simulink model "Sim_tanksmodel_FGS"  (R2020b)
settings: Solver=FixedStepAuto  StartTime=0.0  StopTime=4000  FixedStep=1  RelTol=1e-3  EnableMultiTasking=on
InitFcn:
  | cd ..
  | cd ..
  | 
  | addpath(genpath('Controlador GS-PID'))
  | cd 'Controlador GS-PID\General'
  | inParameters
StopFcn:
  | BestGains1 = [AS(1).Kp AS(1).Ki AS(1).Kd];
  | BestGains2 = [AS(2).Kp AS(2).Ki AS(2).Kd];
  | BestGains3 = [AS(3).Kp AS(3).Ki AS(3).Kd];
  | save('deletetoreset.mat','BestGains1','BestGains2','BestGains3')
  | 
  | BestGains1 = SA(1).BestSol.Gain;
  | BestGains2 = SA(2).BestSol.Gain;
  | BestGains3 = SA(3).BestSol.Gain;
  | save('reset.mat','BestGains1','BestGains2','BestGains3')
undefined symbols (not defined in the file or in its folder): AS, he1, he2, Kd1, Kd2, Kd3, Ki1, Ki2, Ki3, Kp1, Kp2, Kp3, SA, Ts
libraries: simulink x4, pid_lib x1
settings Model: SimulationMode=accelerator  Creator=sahandar  LastModifiedBy=Usuario
settings SolverCC: AlgebraicLoopSolver=LineSearch
settings DataIOCC: LimitDataPoints=on  SaveFormat=Array  ReturnWorkspaceOutputs=off
settings OptimizationCC: LifeSpan=inf
settings DebuggingCC: AllowSymbolicDim=off  SFUnexpectedBacktrackingDiag=warning  SFNoUnconditionalDefaultTransitionDiag=warning  SFExecutionAtInitializationDiag=none  ArithmeticOperatorsInVariantConditions=warning
settings HardwareCC: ProdBitPerPointer=32  ProdBitPerSizeT=32  ProdBitPerPtrDiffT=32  ProdLargestAtomicFloat=None  ProdIntDivRoundTo=Undefined  ProdEndianess=Unspecified  ProdWordSize=32  ProdHWDeviceType=32-bit Generic
settings ModelReferenceCC: PropagateSignalLabelsOutOfModel=off
settings SFSimCC: SimUseLocalCustomCode=off  CustomCodeUndefinedFunction=UseInterfaceOnly
settings RTWCC: RTWUseLocalCustomCode=off
settings CodeAppCC: StateflowObjectComments=on
settings GRTTargetCC: TargetLangStandard=C89/C90 (ANSI)
settings ConfigComp: CovMetricSettings=dw  CovSaveCumulativeToWorkspaceVar=on  CovSaveSingleToWorkspaceVar=on  CovExternalEMLEnable=off

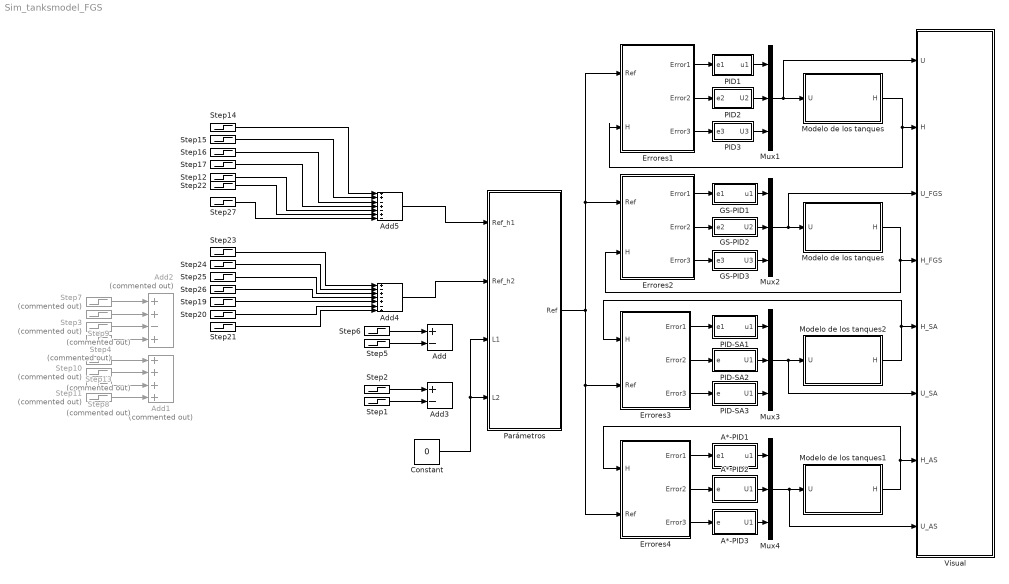
== system Sim_tanksmodel_FGS ==
  A*-PID1 : Subsystem
  A*-PID2 : Subsystem
  A*-PID3 : Subsystem
  Add : Sum  Inputs=+-
  Add1 : Sum  Commented=on  Inputs=++++
  Add2 : Sum  Commented=on  Inputs=++-+
  Add3 : Sum  Inputs=+-
  Add4 : Sum  Inputs=+-+-+-+
  Add5 : Sum  Inputs=++-+-+-
  Constant : Constant  Value=0
  Errores1 : Subsystem
  Errores2 : Subsystem
  Errores3 : Subsystem
  Errores4 : Subsystem
  GS-PID1 : Subsystem
  GS-PID2 : Subsystem
  GS-PID3 : Subsystem
  Modelo de los tanques : Subsystem
  "Modelo de los tanques " : Subsystem
  Modelo de los tanques1 : Subsystem
  Modelo de los tanques2 : Subsystem
  Mux{1..4} (4 alike) : Mux  Inputs=3
  PID-SA1 : Subsystem
  PID-SA2 : Subsystem
  PID-SA3 : Subsystem
  PID1 : Subsystem
  PID2 : Subsystem
  PID3 : Subsystem
  Parámetros : Subsystem
  Step1 : Step  Time=900  SampleTime=Ts
  Step10 : Step  Commented=on  Time=350  After=-0.03  SampleTime=Ts
  Step11 : Step  Commented=on  Time=1100  After=-0.03  SampleTime=Ts
  Step12 : Step  Time=2000  After=0.06  SampleTime=Ts
  Step13 : Step  Commented=on  Time=0  Before=he2  After=0.05  SampleTime=Ts
  Step14 : Step  Time=0  Before=he1  After=0.02  SampleTime=Ts
  Step15 : Step  Time=500  After=0.06  SampleTime=Ts
  Step16 : Step  Time=1000  After=0.06  SampleTime=Ts
  Step17 : Step  Time=1500  After=0.06  SampleTime=Ts
  Step19 : Step  Time=2000  After=0.06  SampleTime=Ts
  Step2 : Step  Time=800  SampleTime=Ts
  Step20 : Step  Time=2500  After=0.06  SampleTime=Ts
  Step21 : Step  Time=3000  After=0.06  SampleTime=Ts
  Step22 : Step  Time=2500  After=0.06  SampleTime=Ts
  Step23 : Step  Time=0  Before=he1  After=0.08  SampleTime=Ts
  Step24 : Step  Time=500  After=0.06  SampleTime=Ts
  Step25 : Step  Time=1000  After=0.06  SampleTime=Ts
  Step26 : Step  Time=1500  After=0.06  SampleTime=Ts
  Step27 : Step  Time=3000  After=0.06  SampleTime=Ts
  Step3 : Step  Commented=on  Time=700  After=0.05  SampleTime=Ts
  Step4 : Step  Commented=on  Time=1100  After=0.05  SampleTime=Ts
  Step5 : Step  Time=800  SampleTime=Ts
  Step6 : Step  Time=600  SampleTime=Ts
  Step7 : Step  Commented=on  Time=0  Before=he1  After=0.15  SampleTime=Ts
  Step8 : Step  Commented=on  Time=700  After=0.02  SampleTime=Ts
  Step9 : Step  Commented=on  Time=350  After=0.05  SampleTime=Ts
  Visual : Subsystem
  wires:
  Mux1/1 -> Modelo de los tanques/1(U), Visual/1(U)
  Modelo de los tanques/1(H) -> Errores1/2(H), Visual/2(H)
  GS-PID3/1(U3) -> Mux2/3
  Errores2/3(Error3) -> GS-PID3/1(e3)
  GS-PID2/1(U2) -> Mux2/2
  Errores2/2(Error2) -> GS-PID2/1(e2)
  GS-PID1/1(u1) -> Mux2/1
  Errores2/1(Error1) -> GS-PID1/1(e1)
  "Modelo de los tanques "/1(H) -> Errores2/2(H), Visual/4(H_FGS)
  Mux2/1 -> Visual/3(U_FGS), "Modelo de los tanques "/1(U)
  PID2/1(U2) -> Mux1/2
  PID3/1(U3) -> Mux1/3
  Errores1/2(Error2) -> PID2/1(e2)
  Errores1/3(Error3) -> PID3/1(e3)
  Errores1/1(Error1) -> PID1/1(e1)
  PID1/1(u1) -> Mux1/1
  PID-SA3/1(U1) -> Mux3/3
  PID-SA2/1(U1) -> Mux3/2
  Modelo de los tanques2/1(H) -> Errores3/1(H), Visual/5(H_SA)
  PID-SA1/1(u1) -> Mux3/1
  Errores3/3(Error3) -> PID-SA3/1(e)
  Errores3/1(Error1) -> PID-SA1/1(e1)
  Errores3/2(Error2) -> PID-SA2/1(e)
  Mux3/1 -> Visual/6(U_SA), Modelo de los tanques2/1(U)
  A*-PID3/1(U1) -> Mux4/3
  Parámetros/1(Ref) -> Errores1/1(Ref), Errores2/1(Ref), Errores3/2(Ref), Errores4/2(Ref)
  A*-PID2/1(U1) -> Mux4/2
  Errores4/2(Error2) -> A*-PID2/1(e)
  A*-PID1/1(u1) -> Mux4/1
  Errores4/3(Error3) -> A*-PID3/1(e)
  Modelo de los tanques1/1(H) -> Errores4/1(H), Visual/7(H_AS)
  Mux4/1 -> Modelo de los tanques1/1(U), Visual/8(U_AS)
  Errores4/1(Error1) -> A*-PID1/1(e1)
  Step3/1 -> Add2/3
  Step8/1 -> Add1/3
  Step9/1 -> Add2/2
  Step4/1 -> Add2/4
  Step7/1 -> Add2/1
  Step13/1 -> Add1/1
  Step11/1 -> Add1/4
  Step5/1 -> Add/2
  Step1/1 -> Add3/2
  Step10/1 -> Add1/2
  Step6/1 -> Add/1
  Step2/1 -> Add3/1
  Constant/1 -> Parámetros/4(L2), Parámetros/3(L1)
  Step24/1 -> Add4/2
  Step26/1 -> Add4/4
  Step19/1 -> Add4/5
  Step25/1 -> Add4/3
  Step14/1 -> Add5/1
  Step27/1 -> Add5/7
  Step23/1 -> Add4/1
  Step17/1 -> Add5/4
  Step20/1 -> Add4/6
  Step12/1 -> Add5/5
  Step22/1 -> Add5/6
  Step21/1 -> Add4/7
  Step16/1 -> Add5/3
  Step15/1 -> Add5/2
  Add5/1 -> Parámetros/1(Ref_h1)
  Add4/1 -> Parámetros/2(Ref_h2)

== system Sim_tanksmodel_FGS/A*-PID1 ==
  e1 : Inport
  Demux : Demux  Outputs=3
  Mux : Mux
  PID Controller : Subsystem
  S-Function : S-Function  FunctionName=sfun_Astar  Parameters=AS_vars1  SFunctionDeploymentMode=off  EnableBusSupport=off
  Saturation1 : Saturate  UpperLimit=1  LowerLimit=0
  Subsystem : Subsystem
  u1 : Outport
  wires:
  Saturation1/1 -> u1/1
  PID Controller/1(u) -> Saturation1/1
  Mux/1 -> S-Function/1
  Subsystem/1(ref) -> Mux/2
  Subsystem/2(enable) -> Mux/3
  S-Function/1 -> Demux/1
  Demux/3 -> PID Controller/4(Kd)  "Kd"
  e1/1 -> PID Controller/1(e), Mux/1
  Subsystem/3(iter) -> Mux/4
  Demux/1 -> PID Controller/2(Kp)  "Kp"
  Demux/2 -> PID Controller/3(Ki)  "Ki"

== system Sim_tanksmodel_FGS/A*-PID2 ==
  e : Inport
  Demux : Demux  Outputs=3
  Mux : Mux
  PID Controller : Subsystem
  S-Function : S-Function  FunctionName=sfun_Astar  Parameters=AS_vars2  SFunctionDeploymentMode=off  EnableBusSupport=off
  Saturation1 : Saturate  UpperLimit=1  LowerLimit=0
  Scope : Scope  NumInputPorts=3
  Subsystem : Subsystem
  U1 : Outport
  wires:
  Demux/2 -> PID Controller/3(Ki), Scope/2  "Ki"
  Demux/1 -> PID Controller/2(Kp), Scope/1  "Kp"
  Subsystem/3(iter) -> Mux/4
  e/1 -> PID Controller/1(e), Mux/1
  Demux/3 -> PID Controller/4(Kd), Scope/3  "Kd"
  S-Function/1 -> Demux/1
  Subsystem/2(enable) -> Mux/3
  Subsystem/1(ref) -> Mux/2
  Mux/1 -> S-Function/1
  Saturation1/1 -> U1/1
  PID Controller/1(u) -> Saturation1/1

== system Sim_tanksmodel_FGS/A*-PID3 ==
  e : Inport
  Demux : Demux  Outputs=3
  Gain : Gain  Gain=-1
  Mux : Mux
  PID Controller : Subsystem
  S-Function : S-Function  FunctionName=sfun_Astar  Parameters=AS_vars3  SFunctionDeploymentMode=off  EnableBusSupport=off
  Saturation1 : Saturate  UpperLimit=1  LowerLimit=0
  Scope : Scope  NumInputPorts=3
  Subsystem : Subsystem
  U1 : Outport
  wires:
  Saturation1/1 -> U1/1
  Mux/1 -> S-Function/1
  Subsystem/1(ref) -> Mux/2
  Subsystem/2(enable) -> Mux/3
  S-Function/1 -> Demux/1
  Demux/3 -> Scope/3, PID Controller/4(Kd)  "Kd"
  e/1 -> Mux/1, PID Controller/1(e)
  Subsystem/3(iter) -> Mux/4
  Demux/1 -> Scope/1, PID Controller/2(Kp)  "Kp"
  Demux/2 -> Scope/2, PID Controller/3(Ki)  "Ki"
  PID Controller/1(u) -> Gain/1
  Gain/1 -> Saturation1/1

== system Sim_tanksmodel_FGS/Errores1 ==
  Ref : Inport
  H : Inport  Port=2
  Add : Sum  Inputs=+-
  Add1 : Sum  Inputs=+-
  Add4 : Sum  Inputs=-+
  Demux : Demux  Outputs=2
  Demux1 : Demux  Outputs=2
  Error1 : Outport
  Error2 : Outport  Port=2
  Error3 : Outport  Port=3
  wires:
  Ref/1 -> Demux/1
  Demux1/2 -> Add1/2  "h2"
  Demux1/1 -> Add/2  "h1"
  Demux/2 -> Add1/1  "ref_h2"
  H/1 -> Demux1/1
  Demux/1 -> Add/1  "ref_h1"
  Add/1 -> Add4/1, Error1/1
  Add1/1 -> Add4/2, Error3/1
  Add4/1 -> Error2/1

== system Sim_tanksmodel_FGS/Errores2 ==
  Ref : Inport
  H : Inport  Port=2
  Add : Sum  Inputs=+-
  Add1 : Sum  Inputs=+-
  Add4 : Sum  Inputs=-+
  Demux : Demux  Outputs=2
  Demux1 : Demux  Outputs=2
  Error1 : Outport
  Error2 : Outport  Port=2
  Error3 : Outport  Port=3
  wires:
  Demux1/2 -> Add1/2  "h2"
  Demux1/1 -> Add/2  "h1"
  Ref/1 -> Demux/1
  Demux/1 -> Add/1  "ref_h1"
  Add1/1 -> Add4/2, Error3/1
  Add4/1 -> Error2/1
  H/1 -> Demux1/1
  Add/1 -> Add4/1, Error1/1
  Demux/2 -> Add1/1  "ref_h2"

== system Sim_tanksmodel_FGS/Errores3 ==
  H : Inport
  Ref : Inport  Port=2
  Add : Sum  Inputs=+-
  Add1 : Sum  Inputs=+-
  Add4 : Sum  Inputs=-+
  Demux : Demux  Outputs=2
  Demux1 : Demux  Outputs=2
  Error1 : Outport
  Error2 : Outport  Port=2
  Error3 : Outport  Port=3
  wires:
  Demux/2 -> Add1/1  "ref_h2"
  Add1/1 -> Add4/2, Error3/1
  Add4/1 -> Error2/1
  H/1 -> Demux1/1
  Add/1 -> Add4/1, Error1/1
  Demux/1 -> Add/1  "ref_h1"
  Demux1/1 -> Add/2  "h1"
  Demux1/2 -> Add1/2  "h2"
  Ref/1 -> Demux/1

== system Sim_tanksmodel_FGS/Errores4 ==
  H : Inport
  Ref : Inport  Port=2
  Add : Sum  Inputs=+-
  Add1 : Sum  Inputs=+-
  Add4 : Sum  Inputs=-+
  Demux : Demux  Outputs=2
  Demux1 : Demux  Outputs=2
  Error1 : Outport
  Error2 : Outport  Port=2
  Error3 : Outport  Port=3
  wires:
  Add4/1 -> Error2/1
  H/1 -> Demux1/1
  Demux/1 -> Add/1  "ref_h1"
  Demux1/1 -> Add/2  "h1"
  Add/1 -> Add4/1, Error1/1
  Demux1/2 -> Add1/2  "h2"
  Add1/1 -> Add4/2, Error3/1
  Demux/2 -> Add1/1  "ref_h2"
  Ref/1 -> Demux/1

== system Sim_tanksmodel_FGS/GS-PID1 ==
  e1 : Inport
  Demux : Demux  Outputs=3
  Divide : Product  Inputs=*/
  Mux : Mux  Inputs=2
  PID Controller : Subsystem
  S-Function1 : S-Function  FunctionName=sfun_fuzzycontrol  Parameters=range_gains1  SFunctionDeploymentMode=off  EnableBusSupport=off
  Saturation1 : Saturate  UpperLimit=1  LowerLimit=0
  Saturation2 : Saturate  UpperLimit=1  LowerLimit=-1
  Saturation3 : Saturate  UpperLimit=1  LowerLimit=-1
  Sum : Sum  Inputs=+-|
  Unit Delay : UnitDelay  SampleTime=-1
  u1 : Outport
  wires:
  Unit Delay/1 -> Sum/2
  Mux/1 -> S-Function1/1
  S-Function1/1 -> Demux/1
  Saturation1/1 -> u1/1
  Demux/1 -> PID Controller/2(Kp)
  Demux/3 -> PID Controller/4(Kd)
  PID Controller/1(u) -> Saturation1/1
  Demux/2 -> PID Controller/3(Ki)
  Saturation2/1 -> Mux/1
  Saturation3/1 -> Mux/2
  e1/1 -> PID Controller/1(e), Divide/1
  Sum/1 -> Saturation3/1
  Divide/1 -> Unit Delay/1, Saturation2/1, Sum/1
  [ref_h1] -> Divide/2

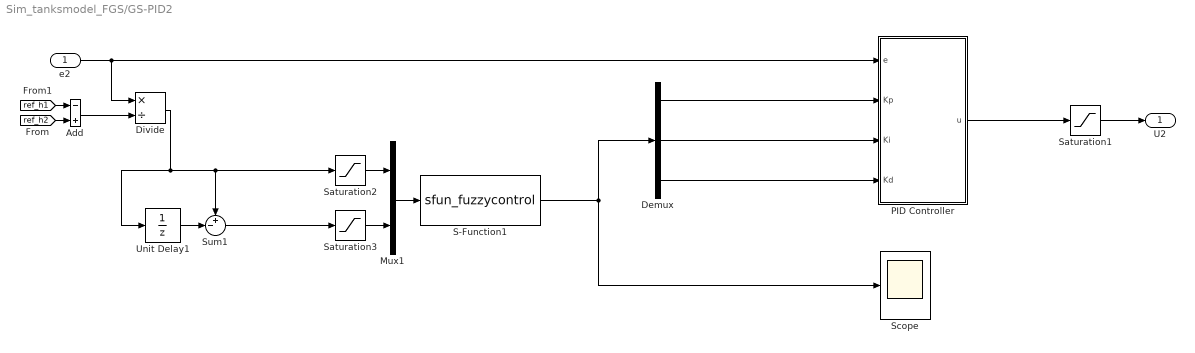
== system Sim_tanksmodel_FGS/GS-PID2 ==
  e2 : Inport
  Add : Sum  Inputs=-+
  Demux : Demux  Outputs=3
  Divide : Product  Inputs=*/
  Mux1 : Mux  Inputs=2
  PID Controller : Subsystem
  S-Function1 : S-Function  FunctionName=sfun_fuzzycontrol  Parameters=range_gains2  SFunctionDeploymentMode=off  EnableBusSupport=off
  Saturation1 : Saturate  UpperLimit=1  LowerLimit=0
  Saturation2 : Saturate  UpperLimit=1  LowerLimit=-1
  Saturation3 : Saturate  UpperLimit=1  LowerLimit=-1
  Scope : Scope
  Sum1 : Sum  Inputs=+-|
  Unit Delay1 : UnitDelay  SampleTime=-1
  U2 : Outport
  wires:
  Demux/2 -> PID Controller/3(Ki)
  Demux/1 -> PID Controller/2(Kp)
  Demux/3 -> PID Controller/4(Kd)
  Saturation1/1 -> U2/1
  S-Function1/1 -> Demux/1, Scope/1
  PID Controller/1(u) -> Saturation1/1
  Unit Delay1/1 -> Sum1/2
  Mux1/1 -> S-Function1/1
  Saturation3/1 -> Mux1/2
  Saturation2/1 -> Mux1/1
  e2/1 -> PID Controller/1(e), Divide/1
  Sum1/1 -> Saturation3/1
  Divide/1 -> Unit Delay1/1, Saturation2/1, Sum1/1
  [ref_h1] -> Add/1
  [ref_h2] -> Add/2
  Add/1 -> Divide/2

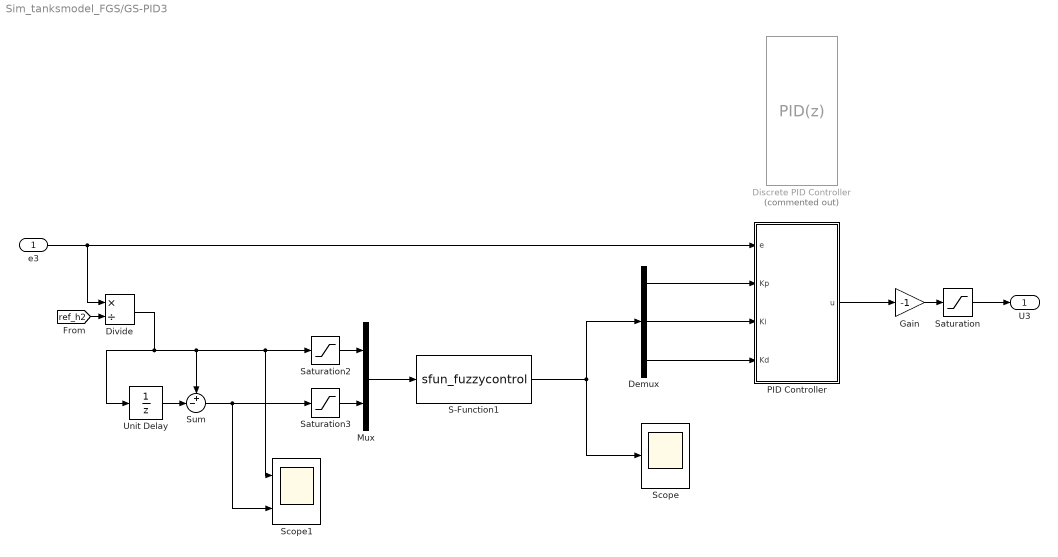
== system Sim_tanksmodel_FGS/GS-PID3 ==
  e3 : Inport
  Demux : Demux  Outputs=3
  Discrete PID Controller : pid_lib/PID Controller  Commented=on  Controller=PID  Form=Parallel  TimeDomain=Discrete-time  UseExternalTs=off  SampleTime=-1  IntegratorMethod=Forward Euler  FilterMethod=Forward Euler  ControllerParametersSource=external  P=1  I=1  D=0  UseFilter=off  N=100  TunerSelectOption=Transfer Function Based (PID Tuner App)  InitialConditionSource=internal  InitialConditionForIntegrator=0  InitialConditionForFilter=0  DifferentiatorICPrevScaledInput=0  ExternalReset=none  TrackingMode=off  Kt=1  LimitOutput=off  SatLimitsSource=internal  UpperSaturationLimit=inf  LowerSaturationLimit=-inf  LinearizeAsGain=off  AntiWindupMode=none  Kb=1  POutMin=[]  POutMax=[]  IOutMin=[]  IOutMax=[]  DOutMin=[]  DOutMax=[]  NOutMin=[]  NOutMax=[]  SumOutMin=[]  SumOutMax=[]  SaturationOutMin=[]  SaturationOutMax=[]  PParamMin=[]  PParamMax=[]  IParamMin=[]  IParamMax=[]  DParamMin=[]  DParamMax=[]  NParamMin=[]  NParamMax=[]  KbParamMin=[]  KbParamMax=[]  KtParamMin=[]  KtParamMax=[]  KbOutMin=[]  KbOutMax=[]  KtOutMin=[]  KtOutMax=[]  IntegratorOutMin=[]  IntegratorOutMax=[]  FilterOutMin=[]  FilterOutMax=[]  SumI1OutMin=[]  SumI1OutMax=[]  SumI2OutMin=[]  SumI2OutMax=[]  SumI3OutMin=[]  SumI3OutMax=[]  SumI4OutMin=[]  SumI4OutMax=[]  SumDOutMin=[]  SumDOutMax=[]  DifferentiatorOutMin=[]  DifferentiatorOutMax=[]  FilterDiffOutCoefMin=[]  FilterDiffOutCoefMax=[]  ReciprocalOutMin=[]  ReciprocalOutMax=[]  SumDenOutMin=[]  SumDenOutMax=[]  SumNumOutMin=[]  SumNumOutMax=[]  DivideOutMin=[]  DivideOutMax=[]  UdiffTsProdOutMin=[]  UdiffTsProdOutMax=[]  NTsProdOutMin=[]  NTsProdOutMax=[]  UintegralTsProdOutMin=[]  UintegralTsProdOutMax=[]  UngainTsProdOutMin=[]  UngainTsProdOutMax=[]  IntegratorContinuousStateAttributes=''  IntegratorStateMustResolveToSignalObject=off  IntegratorRTWStateStorageClass=Auto  FilterContinuousStateAttributes=''  FilterStateMustResolveToSignalObject=off  FilterRTWStateStorageClass=Auto  ParallelPVariant=ExternalParameters  IdealPVariant=Disabled  IVariant=ExternalParameters  DVariant=ExternalParameters  IntegratorVariant=Discrete  SatVariant=Disabled  AWVariant=Passthrough  PCopyVariant=Disabled  TRVariant=Disabled  FdbkBlocksVariant=Forward  IdealPFdbkVariant=Disabled  SatFdbkVariant=Disabled  DerivativeFilterVariant=Differentiator  NVariant=Passthrough  NCopyVariant=Disabled_SignalSpec  FilterICVariant=InternalICsDifferentiator  IntegratorICVariant=InternalICs  ExternalResetVariant=Disabled  TRSumVariant=Passthrough  SumFdbkVariant=Disabled  SumVariant=Sum_PID  TsampFilterVariant=InternalTs  TsampNgainVariant=Passthrough  TsampIntegralVariant=Passthrough  ExternalSaturationOutDataTypeStr=Inherit: Same as second input
  Divide : Product  Inputs=*/
  Gain : Gain  Gain=-1
  Mux : Mux  Inputs=2
  PID Controller : Subsystem
  S-Function1 : S-Function  FunctionName=sfun_fuzzycontrol  Parameters=range_gains3  SFunctionDeploymentMode=off  EnableBusSupport=off
  Saturation : Saturate  UpperLimit=1  LowerLimit=0
  Saturation2 : Saturate  UpperLimit=1  LowerLimit=-1
  Saturation3 : Saturate  UpperLimit=1  LowerLimit=-1
  Scope : Scope
  Scope1 : Scope  NumInputPorts=2
  Sum : Sum  Inputs=+-|
  Unit Delay : UnitDelay  SampleTime=-1
  U3 : Outport
  wires:
  Demux/2 -> PID Controller/3(Ki)
  Demux/1 -> PID Controller/2(Kp)
  Demux/3 -> PID Controller/4(Kd)
  Saturation/1 -> U3/1
  S-Function1/1 -> Demux/1, Scope/1
  Gain/1 -> Saturation/1
  PID Controller/1(u) -> Gain/1
  Unit Delay/1 -> Sum/2
  Mux/1 -> S-Function1/1
  Saturation3/1 -> Mux/2
  Saturation2/1 -> Mux/1
  e3/1 -> PID Controller/1(e), Divide/1
  Sum/1 -> Scope1/2, Saturation3/1
  Divide/1 -> Scope1/1, Saturation2/1, Sum/1, Unit Delay/1
  [ref_h2] -> Divide/2

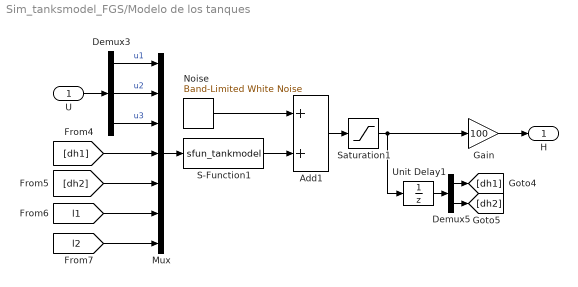
== system Sim_tanksmodel_FGS/Modelo de los tanques ==
  U : Inport
  Add1 : Sum
  Demux3 : Demux  Outputs=3
  Demux5 : Demux  Outputs=2
  Gain : Gain  Gain=100
  Mux : Mux  Inputs=7
  Noise : simulink/Sources/Band-Limited White Noise  Cov=N  Ts=Ts  seed=[23341]
  S-Function1 : S-Function  FunctionName=sfun_tankmodel  Parameters=vars  SFunctionDeploymentMode=off  EnableBusSupport=off
  Saturation1 : Saturate  UpperLimit=25  LowerLimit=0
  Unit Delay1 : UnitDelay  SampleTime=-1  HasFrameUpgradeWarning=on
  H : Outport  VectorParamsAs1DForOutWhenUnconnected=off
  wires:
  Saturation1/1 -> Gain/1, Unit Delay1/1
  Demux3/2 -> Mux/2  "u2"
  Noise/1 -> Add1/1
  [l2] -> Mux/7
  [l1] -> Mux/6
  S-Function1/1 -> Add1/2
  [dh2] -> Mux/5
  Demux3/3 -> Mux/3  "u3"
  Add1/1 -> Saturation1/1
  U/1 -> Demux3/1
  Demux3/1 -> Mux/1  "u1"
  [dh1] -> Mux/4
  Mux/1 -> S-Function1/1
  Gain/1 -> H/1
  Unit Delay1/1 -> Demux5/1
  Demux5/1 -> [dh1]
  Demux5/2 -> [dh2]

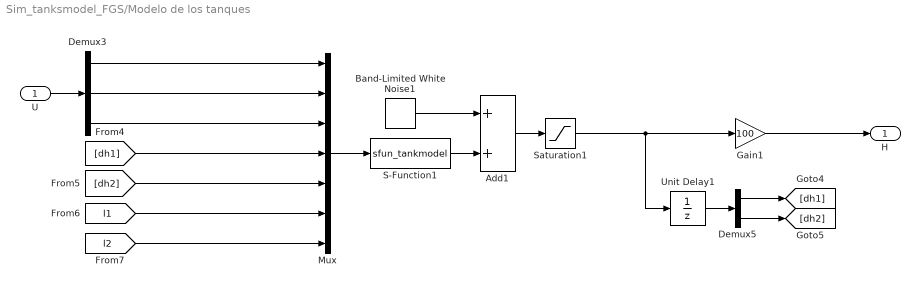
== system Sim_tanksmodel_FGS/Modelo de los tanques  ==
  U : Inport
  Add1 : Sum
  Band-Limited White Noise1 : simulink/Sources/Band-Limited White Noise  Cov=N  Ts=Ts  seed=[23341]
  Demux3 : Demux  Outputs=3
  Demux5 : Demux  Outputs=2
  Gain1 : Gain  Gain=100
  Mux : Mux  Inputs=7
  S-Function1 : S-Function  FunctionName=sfun_tankmodel  Parameters=vars  SFunctionDeploymentMode=off  EnableBusSupport=off
  Saturation1 : Saturate  UpperLimit=inf  LowerLimit=0
  Unit Delay1 : UnitDelay  SampleTime=-1  HasFrameUpgradeWarning=on
  H : Outport  VectorParamsAs1DForOutWhenUnconnected=off
  wires:
  Demux5/2 -> [dh2]
  Demux5/1 -> [dh1]
  Unit Delay1/1 -> Demux5/1
  Mux/1 -> S-Function1/1
  [dh1] -> Mux/4
  Demux3/1 -> Mux/1
  U/1 -> Demux3/1
  Add1/1 -> Saturation1/1
  Demux3/3 -> Mux/3
  [dh2] -> Mux/5
  S-Function1/1 -> Add1/2
  [l1] -> Mux/6
  [l2] -> Mux/7
  Band-Limited White Noise1/1 -> Add1/1
  Demux3/2 -> Mux/2
  Saturation1/1 -> Gain1/1, Unit Delay1/1
  Gain1/1 -> H/1

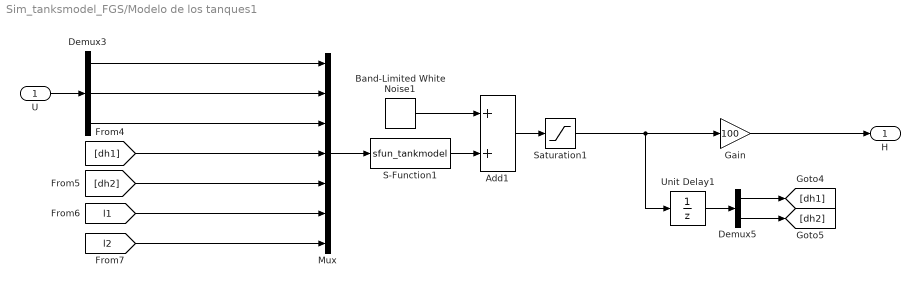
== system Sim_tanksmodel_FGS/Modelo de los tanques1 ==
  U : Inport
  Add1 : Sum
  Band-Limited White Noise1 : simulink/Sources/Band-Limited White Noise  Cov=N  Ts=Ts  seed=[23341]
  Demux3 : Demux  Outputs=3
  Demux5 : Demux  Outputs=2
  Gain : Gain  Gain=100
  Mux : Mux  Inputs=7
  S-Function1 : S-Function  FunctionName=sfun_tankmodel  Parameters=vars  SFunctionDeploymentMode=off  EnableBusSupport=off
  Saturation1 : Saturate  UpperLimit=0.25  LowerLimit=0
  Unit Delay1 : UnitDelay  SampleTime=-1  HasFrameUpgradeWarning=on
  H : Outport  VectorParamsAs1DForOutWhenUnconnected=off
  wires:
  Demux5/2 -> [dh2]
  Demux5/1 -> [dh1]
  Unit Delay1/1 -> Demux5/1
  Mux/1 -> S-Function1/1
  [dh1] -> Mux/4
  Demux3/1 -> Mux/1
  U/1 -> Demux3/1
  Add1/1 -> Saturation1/1
  Demux3/3 -> Mux/3
  [dh2] -> Mux/5
  S-Function1/1 -> Add1/2
  [l1] -> Mux/6
  [l2] -> Mux/7
  Band-Limited White Noise1/1 -> Add1/1
  Demux3/2 -> Mux/2
  Saturation1/1 -> Gain/1, Unit Delay1/1
  Gain/1 -> H/1

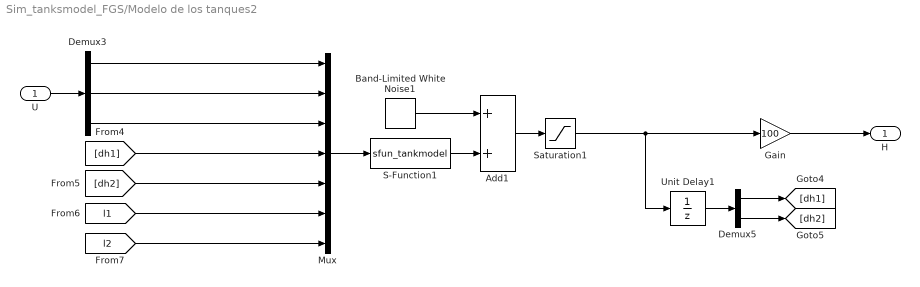
== system Sim_tanksmodel_FGS/Modelo de los tanques2 ==
  U : Inport
  Add1 : Sum
  Band-Limited White Noise1 : simulink/Sources/Band-Limited White Noise  Cov=N  Ts=Ts  seed=[23341]
  Demux3 : Demux  Outputs=3
  Demux5 : Demux  Outputs=2
  Gain : Gain  Gain=100
  Mux : Mux  Inputs=7
  S-Function1 : S-Function  FunctionName=sfun_tankmodel  Parameters=vars  SFunctionDeploymentMode=off  EnableBusSupport=off
  Saturation1 : Saturate  UpperLimit=inf  LowerLimit=0
  Unit Delay1 : UnitDelay  SampleTime=-1  HasFrameUpgradeWarning=on
  H : Outport  VectorParamsAs1DForOutWhenUnconnected=off
  wires:
  Demux5/2 -> [dh2]
  Demux5/1 -> [dh1]
  Unit Delay1/1 -> Demux5/1
  Mux/1 -> S-Function1/1
  [dh1] -> Mux/4
  Demux3/1 -> Mux/1
  U/1 -> Demux3/1
  Add1/1 -> Saturation1/1
  Demux3/3 -> Mux/3
  [dh2] -> Mux/5
  S-Function1/1 -> Add1/2
  [l1] -> Mux/6
  [l2] -> Mux/7
  Band-Limited White Noise1/1 -> Add1/1
  Demux3/2 -> Mux/2
  Saturation1/1 -> Gain/1, Unit Delay1/1
  Gain/1 -> H/1

== system Sim_tanksmodel_FGS/PID-SA1 ==
  e1 : Inport
  Demux : Demux
  Mux : Mux  Inputs=6
  PID Controller : Subsystem
  S-Function : S-Function  FunctionName=sfun_SA  Parameters=SA_vars1  SFunctionDeploymentMode=off  EnableBusSupport=off
  Saturation1 : Saturate  UpperLimit=1  LowerLimit=0
  Subsystem : Subsystem
  Terminator : Terminator
  u1 : Outport
  wires:
  Saturation1/1 -> u1/1
  PID Controller/1(u) -> Saturation1/1
  Mux/1 -> S-Function/1
  Subsystem/1(ref) -> Mux/2
  Subsystem/2(enable) -> Mux/3
  Subsystem/5(Gains_out) -> Mux/6
  Demux/3 -> PID Controller/3(Ki)  "Ki1"
  Demux/2 -> PID Controller/2(Kp)  "Kp1"
  S-Function/1 -> Subsystem/1(Gains_in), Demux/1
  Demux/4 -> PID Controller/4(Kd)  "Kd1"
  e1/1 -> PID Controller/1(e), Mux/1
  Subsystem/3(iter) -> Mux/4
  Subsystem/4(Subiter) -> Mux/5
  Demux/1 -> Terminator/1  "J1"

== system Sim_tanksmodel_FGS/PID-SA2 ==
  e : Inport
  Demux : Demux
  Mux : Mux  Inputs=6
  PID Controller : Subsystem
  S-Function : S-Function  FunctionName=sfun_SA  Parameters=SA_vars2  SFunctionDeploymentMode=off  EnableBusSupport=off
  Saturation1 : Saturate  UpperLimit=1  LowerLimit=0
  Scope : Scope  NumInputPorts=4
  Subsystem : Subsystem
  U1 : Outport
  wires:
  Subsystem/4(Subiter) -> Mux/5
  Subsystem/3(iter) -> Mux/4
  e/1 -> PID Controller/1(e), Mux/1
  Demux/4 -> Scope/4, PID Controller/4(Kd)  "Kd1"
  Demux/1 -> Scope/1  "J1"
  S-Function/1 -> Subsystem/1(Gains_in), Demux/1
  Demux/2 -> Scope/2, PID Controller/2(Kp)  "Kp1"
  Demux/3 -> Scope/3, PID Controller/3(Ki)  "Ki1"
  Subsystem/5(Gains_out) -> Mux/6
  Subsystem/2(enable) -> Mux/3
  Subsystem/1(ref) -> Mux/2
  Mux/1 -> S-Function/1
  PID Controller/1(u) -> Saturation1/1
  Saturation1/1 -> U1/1

== system Sim_tanksmodel_FGS/PID-SA3 ==
  e : Inport
  Demux : Demux
  Gain : Gain  Gain=-1
  Mux : Mux  Inputs=6
  PID Controller : Subsystem
  S-Function : S-Function  FunctionName=sfun_SA  Parameters=SA_vars3  SFunctionDeploymentMode=off  EnableBusSupport=off
  Saturation1 : Saturate  UpperLimit=1  LowerLimit=0
  Scope : Scope  NumInputPorts=4
  Subsystem : Subsystem
  U1 : Outport
  wires:
  Saturation1/1 -> U1/1
  Mux/1 -> S-Function/1
  Subsystem/1(ref) -> Mux/2
  Subsystem/2(enable) -> Mux/3
  Subsystem/5(Gains_out) -> Mux/6
  Demux/3 -> PID Controller/3(Ki), Scope/3  "Ki1"
  Demux/2 -> PID Controller/2(Kp), Scope/2  "Kp1"
  S-Function/1 -> Demux/1, Subsystem/1(Gains_in)
  Demux/1 -> Scope/1  "J1"
  Demux/4 -> PID Controller/4(Kd), Scope/4  "Kd1"
  e/1 -> Mux/1, PID Controller/1(e)
  Subsystem/3(iter) -> Mux/4
  Subsystem/4(Subiter) -> Mux/5
  PID Controller/1(u) -> Gain/1
  Gain/1 -> Saturation1/1

== system Sim_tanksmodel_FGS/PID1 ==
  e1 : Inport
  Constant : Constant  Value=Kp1
  Constant1 : Constant  Value=Ki1
  Constant2 : Constant  Value=Kd1
  PID Controller : Subsystem
  Saturation : Saturate  UpperLimit=1  LowerLimit=0
  u1 : Outport
  wires:
  Constant2/1 -> PID Controller/4(Kd)
  Constant/1 -> PID Controller/2(Kp)
  e1/1 -> PID Controller/1(e)
  Saturation/1 -> u1/1
  PID Controller/1(u) -> Saturation/1
  Constant1/1 -> PID Controller/3(Ki)

== system Sim_tanksmodel_FGS/PID2 ==
  e2 : Inport
  Constant : Constant  Value=Kp2
  Constant1 : Constant  Value=Ki2
  Constant2 : Constant  Value=Kd2
  PID Controller : Subsystem
  Saturation : Saturate  UpperLimit=1  LowerLimit=0
  U2 : Outport
  wires:
  Saturation/1 -> U2/1
  e2/1 -> PID Controller/1(e)
  Constant/1 -> PID Controller/2(Kp)
  Constant1/1 -> PID Controller/3(Ki)
  Constant2/1 -> PID Controller/4(Kd)
  PID Controller/1(u) -> Saturation/1

== system Sim_tanksmodel_FGS/PID3 ==
  e3 : Inport
  Constant : Constant  Value=Kp3
  Constant1 : Constant  Value=Ki3
  Constant2 : Constant  Value=Kd3
  Gain : Gain  Gain=-1
  PID Controller : Subsystem
  Saturation : Saturate  UpperLimit=1  LowerLimit=0
  U3 : Outport
  wires:
  Constant2/1 -> PID Controller/4(Kd)
  Constant1/1 -> PID Controller/3(Ki)
  Constant/1 -> PID Controller/2(Kp)
  e3/1 -> PID Controller/1(e)
  Saturation/1 -> U3/1
  PID Controller/1(u) -> Gain/1
  Gain/1 -> Saturation/1

== system Sim_tanksmodel_FGS/Parámetros ==
  Ref_h1 : Inport
  Ref_h2 : Inport  Port=2
  L1 : Inport  Port=3
  L2 : Inport  Port=4
  Gain1 : Gain  Gain=100
  Gain3 : Gain  Gain=100
  Mux : Mux  Inputs=2
  Ref : Outport
  tag scope: l1=global, l2=global, ref_h1=global, ref_h2=global
  wires:
  L1/1 -> [l1]
  Mux/1 -> Ref/1
  Ref_h1/1 -> Gain3/1
  L2/1 -> [l2]
  Ref_h2/1 -> Gain1/1
  Gain3/1 -> Mux/1, [ref_h1]
  Gain1/1 -> [ref_h2], Mux/2

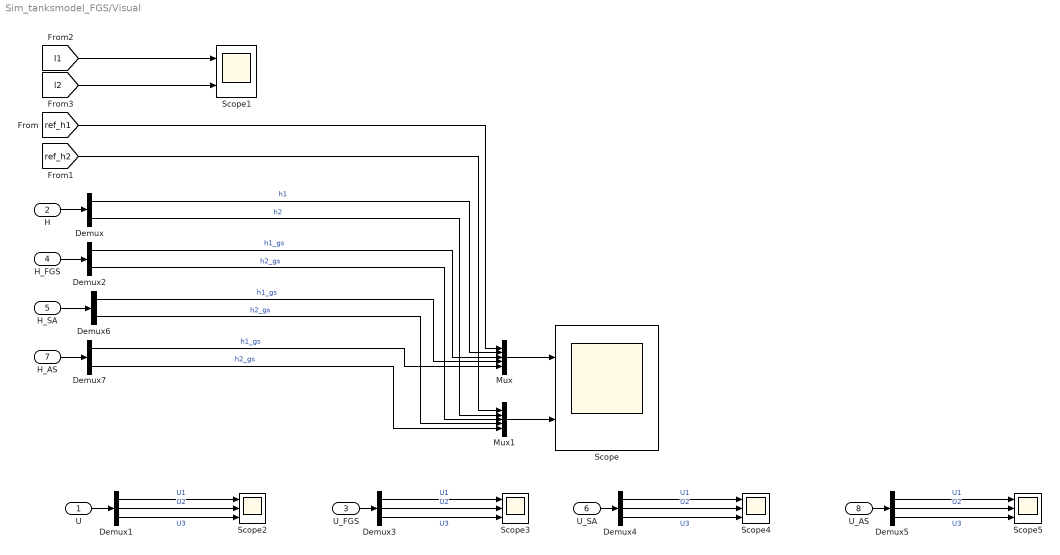
== system Sim_tanksmodel_FGS/Visual ==
  U : Inport
  H : Inport  Port=2
  U_FGS : Inport  Port=3
  H_FGS : Inport  Port=4
  H_SA : Inport  Port=5
  U_SA : Inport  Port=6
  H_AS : Inport  Port=7
  U_AS : Inport  Port=8
  Demux{,2,6..7} (4 alike) : Demux  Outputs=2
  Demux{1,3..5} (4 alike) : Demux  Outputs=3
  Mux : Mux  Inputs=5
  Mux1 : Mux  Inputs=5
  Scope : Scope  NumInputPorts=2
  Scope1 : Scope  NumInputPorts=2
  Scope{2..5} (4 alike) : Scope  NumInputPorts=3
  wires:
  H/1 -> Demux/1
  Demux/1 -> Mux/2  "h1"
  [ref_h1] -> Mux/1
  Mux/1 -> Scope/1
  Demux/2 -> Mux1/2  "h2"
  [ref_h2] -> Mux1/1
  [l1] -> Scope1/1
  [l2] -> Scope1/2
  U/1 -> Demux1/1
  Demux1/1 -> Scope2/1  "U1"
  Demux1/2 -> Scope2/2  "U2"
  Demux1/3 -> Scope2/3  "U3"
  Mux1/1 -> Scope/2
  Demux2/1 -> Mux/3  "h1_gs"
  H_FGS/1 -> Demux2/1
  Demux2/2 -> Mux1/3  "h2_gs"
  Demux3/3 -> Scope3/3  "U3"
  Demux3/2 -> Scope3/2  "U2"
  Demux3/1 -> Scope3/1  "U1"
  U_FGS/1 -> Demux3/1
  U_SA/1 -> Demux4/1
  Demux4/1 -> Scope4/1  "U1"
  Demux4/2 -> Scope4/2  "U2"
  Demux4/3 -> Scope4/3  "U3"
  Demux5/3 -> Scope5/3  "U3"
  Demux5/2 -> Scope5/2  "U2"
  Demux5/1 -> Scope5/1  "U1"
  U_AS/1 -> Demux5/1
  H_SA/1 -> Demux6/1
  H_AS/1 -> Demux7/1
  Demux6/1 -> Mux/4  "h1_gs"
  Demux7/1 -> Mux/5  "h1_gs"
  Demux6/2 -> Mux1/4  "h2_gs"
  Demux7/2 -> Mux1/5  "h2_gs"

== system Sim_tanksmodel_FGS/A*-PID1/PID Controller ==
  e : Inport
  Kp : Inport  Port=2
  Ki : Inport  Port=3
  Kd : Inport  Port=4
  Derivative : Derivative
  Integrator : Integrator
  Product : Product
  Product1 : Product
  Product2 : Product
  Sum : Sum  Inputs=3
  u : Outport
  wires:
  Sum/1 -> u/1
  Product/1 -> Sum/1
  Kp/1 -> Product/2
  Ki/1 -> Product1/2
  Integrator/1 -> Product1/1
  Product1/1 -> Sum/2
  Product2/1 -> Sum/3
  Kd/1 -> Product2/2
  e/1 -> Derivative/1, Integrator/1, Product/1
  Derivative/1 -> Product2/1

== system Sim_tanksmodel_FGS/A*-PID1/Subsystem ==
  Constant1 : Constant  Value=he1
  Constant3 : Constant  Value=AS(1).iter
  Contador : MATLAB Function  TreatAsAtomicUnit=on
  Delay : Delay  DelayLength=1  InitialCondition=0
  Delay3 : Delay  DelayLength=1  InitialCondition=he1
  Delay5 : Delay  DelayLength=1  InitialCondition=0
  Delay6 : Delay  DelayLength=1  InitialCondition=0
  Detector de flancos : MATLAB Function  TreatAsAtomicUnit=on
  Scope5 : Scope  NumInputPorts=3
  ref : Outport
  enable : Outport  Port=2
  iter : Outport  Port=3
  wires:
  Contador/1(iter) -> Delay6/1
  Delay/1 -> Contador/3(u_1)
  [ref_h1] -> Delay3/1, Detector de flancos/2(r), Delay5/1
  Delay3/1 -> Detector de flancos/3(r_1)
  Delay5/1 -> Scope5/1, ref/1
  Delay6/1 -> Scope5/3, iter/1, Contador/4("iter ")
  Detector de flancos/1(signal) -> Delay/1, Contador/2(u), Scope5/2, enable/1
  Constant1/1 -> Detector de flancos/1(he1)
  Constant3/1 -> Contador/1(it_init)

== system Sim_tanksmodel_FGS/A*-PID2/PID Controller ==
  e : Inport
  Kp : Inport  Port=2
  Ki : Inport  Port=3
  Kd : Inport  Port=4
  Derivative : Derivative
  Integrator : Integrator
  Product : Product
  Product1 : Product
  Product2 : Product
  Sum : Sum  Inputs=3
  u : Outport
  wires:
  Derivative/1 -> Product2/1
  e/1 -> Product/1, Integrator/1, Derivative/1
  Kd/1 -> Product2/2
  Product2/1 -> Sum/3
  Product1/1 -> Sum/2
  Integrator/1 -> Product1/1
  Ki/1 -> Product1/2
  Kp/1 -> Product/2
  Product/1 -> Sum/1
  Sum/1 -> u/1

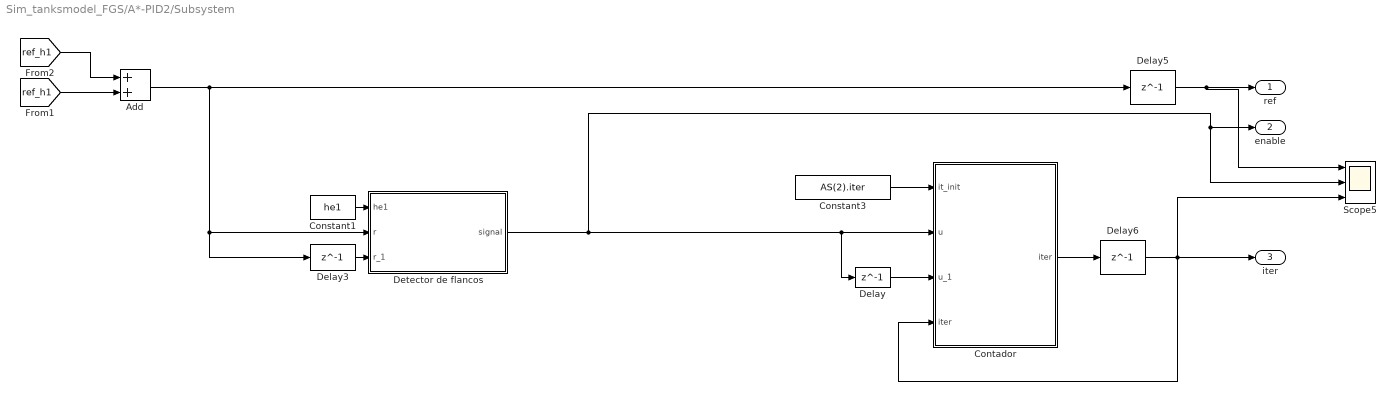
== system Sim_tanksmodel_FGS/A*-PID2/Subsystem ==
  Add : Sum
  Constant1 : Constant  Value=he1
  Constant3 : Constant  Value=AS(2).iter
  Contador : MATLAB Function  TreatAsAtomicUnit=on
  Delay : Delay  DelayLength=1  InitialCondition=0
  Delay3 : Delay  DelayLength=1  InitialCondition=he1
  Delay5 : Delay  DelayLength=1  InitialCondition=0
  Delay6 : Delay  DelayLength=1  InitialCondition=0
  Detector de flancos : MATLAB Function  TreatAsAtomicUnit=on
  Scope5 : Scope  NumInputPorts=3
  ref : Outport
  enable : Outport  Port=2
  iter : Outport  Port=3
  wires:
  Constant3/1 -> Contador/1(it_init)
  Constant1/1 -> Detector de flancos/1(he1)
  Detector de flancos/1(signal) -> enable/1, Scope5/2, Contador/2(u), Delay/1
  Delay6/1 -> Contador/4("iter "), iter/1, Scope5/3
  Delay5/1 -> ref/1, Scope5/1
  Delay3/1 -> Detector de flancos/3(r_1)
  Add/1 -> Delay5/1, Detector de flancos/2(r), Delay3/1
  Delay/1 -> Contador/3(u_1)
  Contador/1(iter) -> Delay6/1
  [ref_h1] -> Add/2
  [ref_h1] -> Add/1

== system Sim_tanksmodel_FGS/A*-PID3/PID Controller ==
  e : Inport
  Kp : Inport  Port=2
  Ki : Inport  Port=3
  Kd : Inport  Port=4
  Derivative : Derivative
  Integrator : Integrator
  Product : Product
  Product1 : Product
  Product2 : Product
  Sum : Sum  Inputs=3
  u : Outport
  wires:
  Sum/1 -> u/1
  Product/1 -> Sum/1
  Kp/1 -> Product/2
  Ki/1 -> Product1/2
  Integrator/1 -> Product1/1
  Product1/1 -> Sum/2
  Product2/1 -> Sum/3
  Kd/1 -> Product2/2
  e/1 -> Derivative/1, Integrator/1, Product/1
  Derivative/1 -> Product2/1

== system Sim_tanksmodel_FGS/A*-PID3/Subsystem ==
  Constant1 : Constant  Value=he1
  Constant3 : Constant  Value=AS(3).iter
  Contador : MATLAB Function  TreatAsAtomicUnit=on
  Delay : Delay  DelayLength=1  InitialCondition=0
  Delay3 : Delay  DelayLength=1  InitialCondition=he1
  Delay5 : Delay  DelayLength=1  InitialCondition=0
  Delay6 : Delay  DelayLength=1  InitialCondition=0
  Detector de flancos : MATLAB Function  TreatAsAtomicUnit=on
  Scope5 : Scope  NumInputPorts=3
  ref : Outport
  enable : Outport  Port=2
  iter : Outport  Port=3
  wires:
  Contador/1(iter) -> Delay6/1
  Delay/1 -> Contador/3(u_1)
  Delay3/1 -> Detector de flancos/3(r_1)
  Delay5/1 -> Scope5/1, ref/1
  Delay6/1 -> Scope5/3, iter/1, Contador/4("iter ")
  Detector de flancos/1(signal) -> Delay/1, Contador/2(u), Scope5/2, enable/1
  Constant1/1 -> Detector de flancos/1(he1)
  Constant3/1 -> Contador/1(it_init)
  [ref_h2] -> Detector de flancos/2(r), Delay3/1, Delay5/1

== system Sim_tanksmodel_FGS/GS-PID1/PID Controller ==
  e : Inport
  Kp : Inport  Port=2
  Ki : Inport  Port=3
  Kd : Inport  Port=4
  Derivative : Derivative
  Integrator : Integrator
  Product : Product
  Product1 : Product
  Product2 : Product
  Sum : Sum  Inputs=3
  u : Outport
  wires:
  Sum/1 -> u/1
  Product/1 -> Sum/1
  Kp/1 -> Product/2
  Ki/1 -> Product1/2
  Integrator/1 -> Product1/1
  Product1/1 -> Sum/2
  Product2/1 -> Sum/3
  Kd/1 -> Product2/2
  e/1 -> Derivative/1, Integrator/1, Product/1
  Derivative/1 -> Product2/1

== system Sim_tanksmodel_FGS/GS-PID2/PID Controller ==
  e : Inport
  Kp : Inport  Port=2
  Ki : Inport  Port=3
  Kd : Inport  Port=4
  Derivative : Derivative
  Integrator : Integrator
  Product : Product
  Product1 : Product
  Product2 : Product
  Sum : Sum  Inputs=3
  u : Outport
  wires:
  Sum/1 -> u/1
  Product/1 -> Sum/1
  Kp/1 -> Product/2
  Ki/1 -> Product1/2
  Integrator/1 -> Product1/1
  Product1/1 -> Sum/2
  Product2/1 -> Sum/3
  Kd/1 -> Product2/2
  e/1 -> Derivative/1, Integrator/1, Product/1
  Derivative/1 -> Product2/1

== system Sim_tanksmodel_FGS/GS-PID3/PID Controller ==
  e : Inport
  Kp : Inport  Port=2
  Ki : Inport  Port=3
  Kd : Inport  Port=4
  Derivative : Derivative
  Integrator : Integrator
  Product : Product
  Product1 : Product
  Product2 : Product
  Sum : Sum  Inputs=3
  u : Outport
  wires:
  Sum/1 -> u/1
  Product/1 -> Sum/1
  Kp/1 -> Product/2
  Ki/1 -> Product1/2
  Integrator/1 -> Product1/1
  Product1/1 -> Sum/2
  Product2/1 -> Sum/3
  Kd/1 -> Product2/2
  e/1 -> Derivative/1, Integrator/1, Product/1
  Derivative/1 -> Product2/1

== system Sim_tanksmodel_FGS/PID-SA1/PID Controller ==
  e : Inport
  Kp : Inport  Port=2
  Ki : Inport  Port=3
  Kd : Inport  Port=4
  Derivative : Derivative
  Integrator : Integrator
  Product : Product
  Product1 : Product
  Product2 : Product
  Sum : Sum  Inputs=3
  u : Outport
  wires:
  Sum/1 -> u/1
  Product/1 -> Sum/1
  Kp/1 -> Product/2
  Ki/1 -> Product1/2
  Integrator/1 -> Product1/1
  Product1/1 -> Sum/2
  Product2/1 -> Sum/3
  Kd/1 -> Product2/2
  e/1 -> Derivative/1, Integrator/1, Product/1
  Derivative/1 -> Product2/1

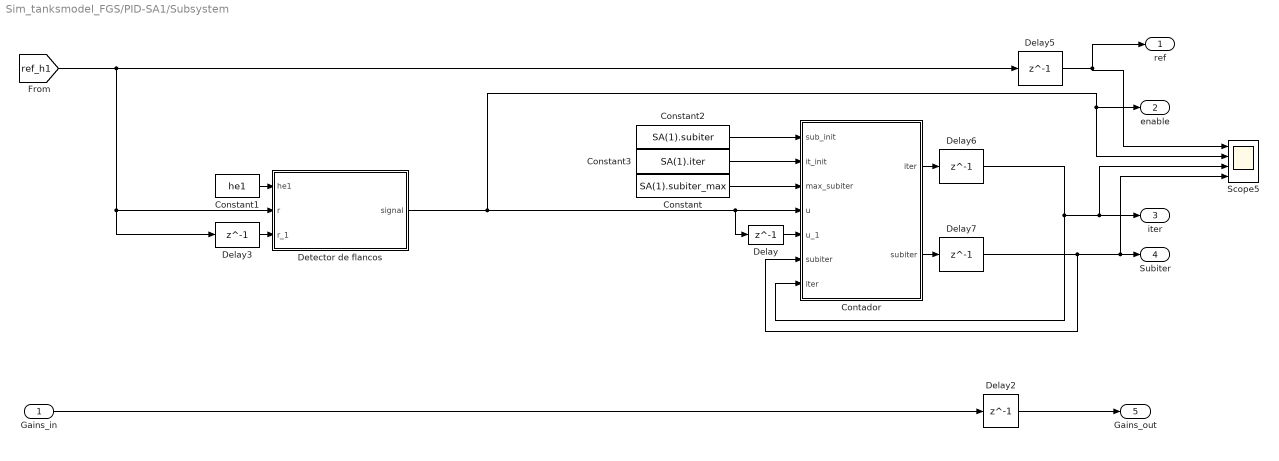
== system Sim_tanksmodel_FGS/PID-SA1/Subsystem ==
  Gains_in : Inport
  Constant : Constant  Value=SA(1).subiter_max
  Constant1 : Constant  Value=he1
  Constant2 : Constant  Value=SA(1).subiter
  Constant3 : Constant  Value=SA(1).iter
  Contador : MATLAB Function  TreatAsAtomicUnit=on
  Delay{,2,5..7} (5 alike) : Delay  DelayLength=1  InitialCondition=0
  Delay3 : Delay  DelayLength=1  InitialCondition=he1
  Detector de flancos : MATLAB Function  TreatAsAtomicUnit=on
  Scope5 : Scope  NumInputPorts=4
  ref : Outport
  enable : Outport  Port=2
  iter : Outport  Port=3
  Subiter : Outport  Port=4
  Gains_out : Outport  Port=5
  wires:
  Contador/1(iter) -> Delay6/1
  Delay/1 -> Contador/5(u_1)
  Gains_in/1 -> Delay2/1
  Delay2/1 -> Gains_out/1
  [ref_h1] -> Delay3/1, Detector de flancos/2(r), Delay5/1
  Delay3/1 -> Detector de flancos/3(r_1)
  Constant/1 -> Contador/3(max_subiter)
  Contador/2(subiter) -> Delay7/1
  Delay5/1 -> Scope5/1, ref/1
  Delay6/1 -> Contador/7("iter "), Scope5/3, iter/1
  Detector de flancos/1(signal) -> Delay/1, Contador/4(u), Scope5/2, enable/1
  Constant1/1 -> Detector de flancos/1(he1)
  Delay7/1 -> Scope5/4, Subiter/1, Contador/6("subiter ")
  Constant2/1 -> Contador/1(sub_init)
  Constant3/1 -> Contador/2(it_init)

== system Sim_tanksmodel_FGS/PID-SA2/PID Controller ==
  e : Inport
  Kp : Inport  Port=2
  Ki : Inport  Port=3
  Kd : Inport  Port=4
  Derivative : Derivative
  Integrator : Integrator
  Product : Product
  Product1 : Product
  Product2 : Product
  Sum : Sum  Inputs=3
  u : Outport
  wires:
  Derivative/1 -> Product2/1
  e/1 -> Product/1, Integrator/1, Derivative/1
  Kd/1 -> Product2/2
  Product2/1 -> Sum/3
  Product1/1 -> Sum/2
  Integrator/1 -> Product1/1
  Ki/1 -> Product1/2
  Kp/1 -> Product/2
  Product/1 -> Sum/1
  Sum/1 -> u/1

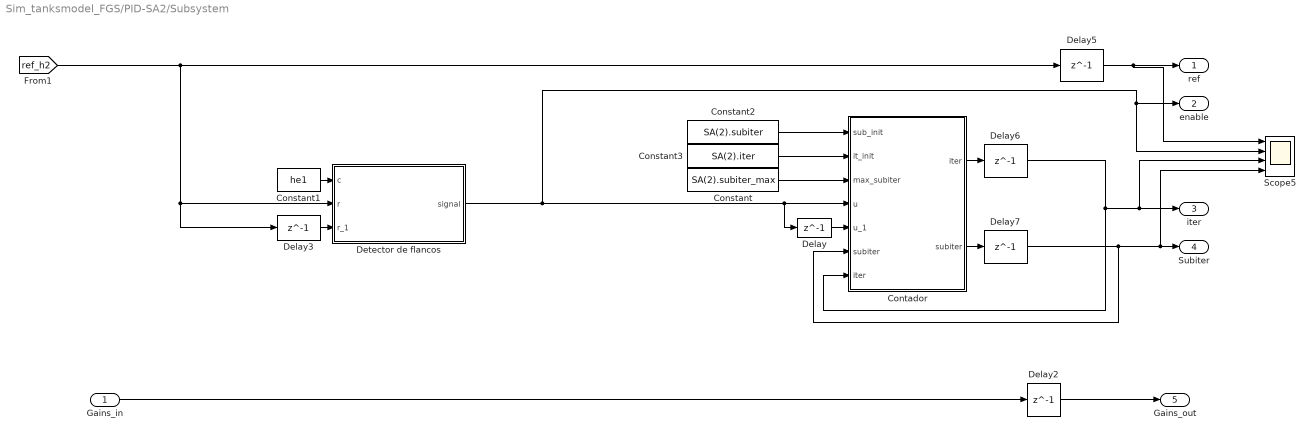
== system Sim_tanksmodel_FGS/PID-SA2/Subsystem ==
  Gains_in : Inport
  Constant : Constant  Value=SA(2).subiter_max
  Constant1 : Constant  Value=he1
  Constant2 : Constant  Value=SA(2).subiter
  Constant3 : Constant  Value=SA(2).iter
  Contador : MATLAB Function  TreatAsAtomicUnit=on
  Delay{,2,5..7} (5 alike) : Delay  DelayLength=1  InitialCondition=0
  Delay3 : Delay  DelayLength=1  InitialCondition=he1
  Detector de flancos : MATLAB Function  TreatAsAtomicUnit=on
  Scope5 : Scope  NumInputPorts=4
  ref : Outport
  enable : Outport  Port=2
  iter : Outport  Port=3
  Subiter : Outport  Port=4
  Gains_out : Outport  Port=5
  wires:
  Constant3/1 -> Contador/2(it_init)
  Constant2/1 -> Contador/1(sub_init)
  Delay7/1 -> Contador/6("subiter "), Subiter/1, Scope5/4
  Constant1/1 -> Detector de flancos/1(c)
  Detector de flancos/1(signal) -> enable/1, Scope5/2, Contador/4(u), Delay/1
  Delay6/1 -> iter/1, Scope5/3, Contador/7("iter ")
  Delay5/1 -> ref/1, Scope5/1
  Contador/2(subiter) -> Delay7/1
  Constant/1 -> Contador/3(max_subiter)
  Delay3/1 -> Detector de flancos/3(r_1)
  [ref_h2] -> Detector de flancos/2(r), Delay3/1, Delay5/1
  Delay2/1 -> Gains_out/1
  Gains_in/1 -> Delay2/1
  Delay/1 -> Contador/5(u_1)
  Contador/1(iter) -> Delay6/1

== system Sim_tanksmodel_FGS/PID-SA3/PID Controller ==
  e : Inport
  Kp : Inport  Port=2
  Ki : Inport  Port=3
  Kd : Inport  Port=4
  Derivative : Derivative
  Integrator : Integrator
  Product : Product
  Product1 : Product
  Product2 : Product
  Sum : Sum  Inputs=3
  u : Outport
  wires:
  Sum/1 -> u/1
  Product/1 -> Sum/1
  Kp/1 -> Product/2
  Ki/1 -> Product1/2
  Integrator/1 -> Product1/1
  Product1/1 -> Sum/2
  Product2/1 -> Sum/3
  Kd/1 -> Product2/2
  e/1 -> Derivative/1, Integrator/1, Product/1
  Derivative/1 -> Product2/1

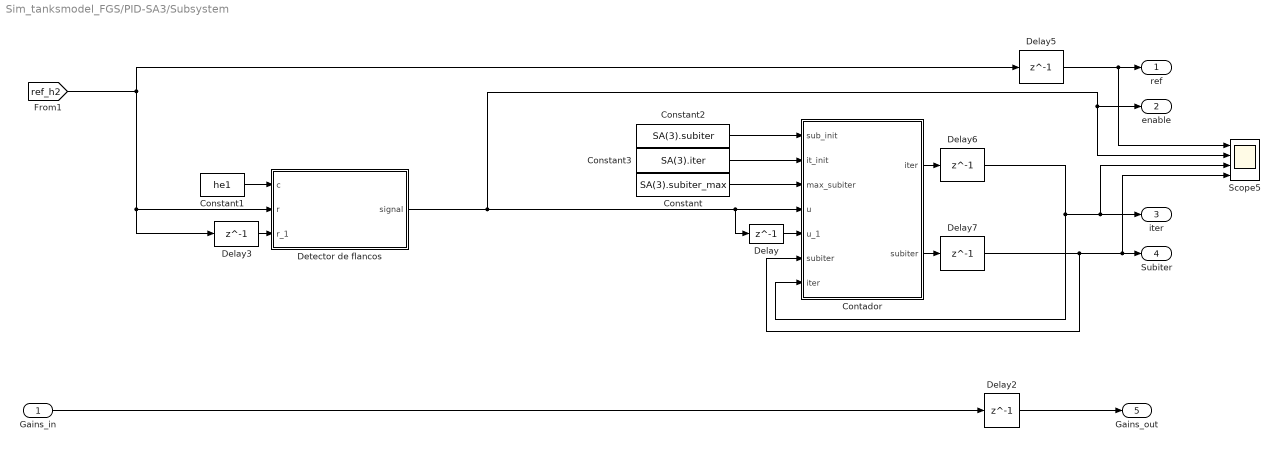
== system Sim_tanksmodel_FGS/PID-SA3/Subsystem ==
  Gains_in : Inport
  Constant : Constant  Value=SA(3).subiter_max
  Constant1 : Constant  Value=he1
  Constant2 : Constant  Value=SA(3).subiter
  Constant3 : Constant  Value=SA(3).iter
  Contador : MATLAB Function  TreatAsAtomicUnit=on
  Delay{,2,5..7} (5 alike) : Delay  DelayLength=1  InitialCondition=0
  Delay3 : Delay  DelayLength=1  InitialCondition=he1
  Detector de flancos : MATLAB Function  TreatAsAtomicUnit=on
  Scope5 : Scope  NumInputPorts=4
  ref : Outport
  enable : Outport  Port=2
  iter : Outport  Port=3
  Subiter : Outport  Port=4
  Gains_out : Outport  Port=5
  wires:
  Contador/1(iter) -> Delay6/1
  Delay/1 -> Contador/5(u_1)
  Gains_in/1 -> Delay2/1
  Delay2/1 -> Gains_out/1
  Delay3/1 -> Detector de flancos/3(r_1)
  Constant/1 -> Contador/3(max_subiter)
  Contador/2(subiter) -> Delay7/1
  Delay5/1 -> Scope5/1, ref/1
  Delay6/1 -> Contador/7("iter "), Scope5/3, iter/1
  Detector de flancos/1(signal) -> Delay/1, Contador/4(u), Scope5/2, enable/1
  Constant1/1 -> Detector de flancos/1(c)
  Delay7/1 -> Scope5/4, Subiter/1, Contador/6("subiter ")
  Constant2/1 -> Contador/1(sub_init)
  Constant3/1 -> Contador/2(it_init)
  [ref_h2] -> Delay5/1, Detector de flancos/2(r), Delay3/1

== system Sim_tanksmodel_FGS/PID1/PID Controller ==
  e : Inport
  Kp : Inport  Port=2
  Ki : Inport  Port=3
  Kd : Inport  Port=4
  Derivative : Derivative
  Integrator : Integrator
  Product : Product
  Product1 : Product
  Product2 : Product
  Sum : Sum  Inputs=3
  u : Outport
  wires:
  Sum/1 -> u/1
  Product/1 -> Sum/1
  Kp/1 -> Product/2
  Ki/1 -> Product1/2
  Integrator/1 -> Product1/1
  Product1/1 -> Sum/2
  Product2/1 -> Sum/3
  Kd/1 -> Product2/2
  e/1 -> Derivative/1, Integrator/1, Product/1
  Derivative/1 -> Product2/1

== system Sim_tanksmodel_FGS/PID2/PID Controller ==
  e : Inport
  Kp : Inport  Port=2
  Ki : Inport  Port=3
  Kd : Inport  Port=4
  Derivative : Derivative
  Integrator : Integrator
  Product : Product
  Product1 : Product
  Product2 : Product
  Sum : Sum  Inputs=3
  u : Outport
  wires:
  Sum/1 -> u/1
  Product/1 -> Sum/1
  Kp/1 -> Product/2
  Ki/1 -> Product1/2
  Integrator/1 -> Product1/1
  Product1/1 -> Sum/2
  Product2/1 -> Sum/3
  Kd/1 -> Product2/2
  e/1 -> Derivative/1, Integrator/1, Product/1
  Derivative/1 -> Product2/1

== system Sim_tanksmodel_FGS/PID3/PID Controller ==
  e : Inport
  Kp : Inport  Port=2
  Ki : Inport  Port=3
  Kd : Inport  Port=4
  Derivative : Derivative
  Integrator : Integrator
  Product : Product
  Product1 : Product
  Product2 : Product
  Sum : Sum  Inputs=3
  u : Outport
  wires:
  Sum/1 -> u/1
  Product/1 -> Sum/1
  Kp/1 -> Product/2
  Ki/1 -> Product1/2
  Integrator/1 -> Product1/1
  Product1/1 -> Sum/2
  Product2/1 -> Sum/3
  Kd/1 -> Product2/2
  e/1 -> Derivative/1, Integrator/1, Product/1
  Derivative/1 -> Product2/1

== matlab function Sim_tanksmodel_FGS/A*-PID2/Subsystem/Contador ==
  data: it_init input; u input; u_1 input; iter output; iter input
function iter  = fcn(it_init, u,u_1,iter)
if iter == 0
    iter = it_init;
end
if u>u_1
    iter =  iter + 1 ;
end

== matlab function Sim_tanksmodel_FGS/A*-PID2/Subsystem/Detector de flancos ==
  data: he1 input; r input; signal output; r_1 input
function signal = fcn(he1, r,r_1)
y = 0;
if (r~=r_1) && r_1 ~=he1
    y = 1;
end
signal = y;

== matlab function Sim_tanksmodel_FGS/A*-PID3/Subsystem/Contador ==
  data: it_init input; u input; u_1 input; iter output; iter input
function iter  = fcn(it_init, u,u_1,iter)
if iter == 0
    iter = it_init;
end
if u>u_1
    iter =  iter + 1 ;
end

== matlab function Sim_tanksmodel_FGS/A*-PID3/Subsystem/Detector de flancos ==
  data: he1 input; r input; signal output; r_1 input
function signal = fcn(he1, r,r_1)
y = 0;
if (r~=r_1) && r_1 ~=he1
    y = 1;
end
signal = y;

== matlab function Sim_tanksmodel_FGS/PID-SA1/Subsystem/Detector de flancos ==
  data: he1 input; r input; signal output; r_1 input
function signal = fcn(he1, r,r_1)
y = 0;
if (r~=r_1) && r_1 ~=he1
    y = 1;
end
signal = y;

== matlab function Sim_tanksmodel_FGS/PID-SA1/Subsystem/Contador ==
  data: sub_init input; it_init input; max_subiter input; u input; u_1 input; subiter input; iter output; subiter output; iter input
function [iter, subiter] = fcn(sub_init,it_init, max_subiter, u,u_1,subiter, iter)
if subiter == 0
    subiter = sub_init;
    iter = it_init;
end
if u>u_1
    subiter =  subiter + 1 ;
end
if subiter == max_subiter + 1
    subiter = 1;
    iter = iter +1;
end

== matlab function Sim_tanksmodel_FGS/PID-SA2/Subsystem/Contador ==
  data: sub_init input; it_init input; max_subiter input; u input; u_1 input; subiter input; iter output; subiter output; iter input
function [iter, subiter] = fcn(sub_init,it_init, max_subiter, u,u_1,subiter, iter)
if subiter == 0
    subiter = sub_init;
    iter = it_init;
end
if u>u_1
    subiter =  subiter + 1 ;
end
if subiter == max_subiter + 1
    subiter = 1;
    iter = iter +1;
end

== matlab function Sim_tanksmodel_FGS/PID-SA2/Subsystem/Detector de flancos ==
  data: c input; r input; signal output; r_1 input
function signal = fcn(c, r,r_1)
y = 0;
if (r~=r_1) && r_1 ~=c
    y = 1;
end
signal = y;

== matlab function Sim_tanksmodel_FGS/A*-PID1/Subsystem/Contador ==
  data: it_init input; u input; u_1 input; iter output; iter input
function iter  = fcn(it_init, u,u_1,iter)
if iter == 0
    iter = it_init;
end
if u>u_1
    iter =  iter + 1 ;
end

== matlab function Sim_tanksmodel_FGS/A*-PID1/Subsystem/Detector de flancos ==
  data: he1 input; r input; signal output; r_1 input
function signal = fcn(he1, r,r_1)
y = 0;
if (r~=r_1) && r_1 ~=he1
    y = 1;
end
signal = y;

== matlab function Sim_tanksmodel_FGS/PID-SA3/Subsystem/Contador ==
  data: sub_init input; it_init input; max_subiter input; u input; u_1 input; subiter input; iter output; subiter output; iter input
function [iter, subiter] = fcn(sub_init,it_init, max_subiter, u,u_1,subiter, iter)
if subiter == 0
    subiter = sub_init;
    iter = it_init;
end
if u>u_1
    subiter =  subiter + 1 ;
end
if subiter == max_subiter + 1
    subiter = 1;
    iter = iter +1;
end

== matlab function Sim_tanksmodel_FGS/PID-SA3/Subsystem/Detector de flancos ==
  data: c input; r input; signal output; r_1 input
function signal = fcn(c, r,r_1)
y = 0;

if (r~=r_1) && r_1 ~=c
    y = 1;
end
signal = y;
